simulink model "ctrl_student_HIL"  (R2015a)
settings: Solver=ode3  StartTime=0.0  StopTime=inf  FixedStep=0.01  RelTol=1e-3
undefined symbols (not defined in the file): DesiredPath, Elipscenter_radi, eta_dot_ini, K, K1, K2, l1, l2, l3, LAW, lim, lim_2, m, mu, pd, T_initialDP, U_ref
libraries: simulink x1
(part 3 of 4)

== system ctrl_student_HIL/tau to CSE mocell (only use for HIL testing) ==
  tau_d to model : Inport
  integrator reset : Inport  Port=2
  Constant : Constant  Value=eta_dot_ini(1)
  Constant1 : Constant  Value=eta_dot_ini(2)
  Constant2 : Constant  Value=eta_dot_ini(3)
  Demux : Demux  Outputs=3
  N_d : S-Function  Priority=2  FunctionName=NIVeriStandIO  Parameters=width dtype portnum stime stype btype  mask(NI VeriStand Outport){portnum=2, width=-1, stime=-1, dtype=auto, stype=auto, btype=0}
      mask prompts: portnum "Port number:"; width "Port dimensions (-1 for dynamically sized):"; stime "Sample time (-1 for inherited):"; dtype "Data type:"; stype "Signal type:"; btype "Block type:"
      mask help: Use this outport on any level of nested subsystems to allow NI VeriStand software to map signals to it.
      mask init:
      | NIVeriStandIO_init;
      settings: CopyFcn=NIVeriStand_MDL_functions('', 'IO_copy');  DeleteFcn=NIVeriStand_MDL_functions('', 'IO_delete');  MoveFcn=set_param(gcb, 'Mask', 'on');
      mask Callback portnum: NIVeriStand_MDL_functions('', 'IO_setportnum');
      mask TypeOptions dtype: auto | double | single | int8 | uint8 | int16 | uint16 | int32 | uint32 | boolean
      mask Callback dtype: NIVeriStand_MDL_functions('', 'IO_booleansignal');
      mask TypeOptions stype: auto | real | complex
      mask Display:
      | patch([-x x], [-y y], [.90980 .81960 .32156]);
      | plot([xrad -x x xrad], [yrad -y y yrad]);
      | fprintf('NI Out%d', portnum);
  X_d : S-Function  Priority=1  FunctionName=NIVeriStandIO  Parameters=width dtype portnum stime stype btype  mask(NI VeriStand Outport){portnum=1, width=-1, stime=-1, dtype=auto, stype=auto, btype=0}
      mask prompts: portnum "Port number:"; width "Port dimensions (-1 for dynamically sized):"; stime "Sample time (-1 for inherited):"; dtype "Data type:"; stype "Signal type:"; btype "Block type:"
      mask help: Use this outport on any level of nested subsystems to allow NI VeriStand software to map signals to it.
      mask init:
      | NIVeriStandIO_init;
      settings: CopyFcn=NIVeriStand_MDL_functions('', 'IO_copy');  DeleteFcn=NIVeriStand_MDL_functions('', 'IO_delete');  MoveFcn=set_param(gcb, 'Mask', 'on');
      mask Callback portnum: NIVeriStand_MDL_functions('', 'IO_setportnum');
      mask TypeOptions dtype: auto | double | single | int8 | uint8 | int16 | uint16 | int32 | uint32 | boolean
      mask Callback dtype: NIVeriStand_MDL_functions('', 'IO_booleansignal');
      mask TypeOptions stype: auto | real | complex
      mask Display:
      | patch([-x x], [-y y], [.90980 .81960 .32156]);
      | plot([xrad -x x xrad], [yrad -y y yrad]);
      | fprintf('NI Out%d', portnum);
  Y_d : S-Function  Priority=3  FunctionName=NIVeriStandIO  Parameters=width dtype portnum stime stype btype  mask(NI VeriStand Outport){portnum=3, width=-1, stime=-1, dtype=auto, stype=auto, btype=0}
      mask prompts: portnum "Port number:"; width "Port dimensions (-1 for dynamically sized):"; stime "Sample time (-1 for inherited):"; dtype "Data type:"; stype "Signal type:"; btype "Block type:"
      mask help: Use this outport on any level of nested subsystems to allow NI VeriStand software to map signals to it.
      mask init:
      | NIVeriStandIO_init;
      settings: CopyFcn=NIVeriStand_MDL_functions('', 'IO_copy');  DeleteFcn=NIVeriStand_MDL_functions('', 'IO_delete');  MoveFcn=set_param(gcb, 'Mask', 'on');
      mask Callback portnum: NIVeriStand_MDL_functions('', 'IO_setportnum');
      mask TypeOptions dtype: auto | double | single | int8 | uint8 | int16 | uint16 | int32 | uint32 | boolean
      mask Callback dtype: NIVeriStand_MDL_functions('', 'IO_booleansignal');
      mask TypeOptions stype: auto | real | complex
      mask Display:
      | patch([-x x], [-y y], [.90980 .81960 .32156]);
      | plot([xrad -x x xrad], [yrad -y y yrad]);
      | fprintf('NI Out%d', portnum);
  integrator reset model : S-Function  Priority=7  FunctionName=NIVeriStandIO  Parameters=width dtype portnum stime stype btype  mask(NI VeriStand Outport){portnum=7, width=-1, stime=-1, dtype=auto, stype=auto, btype=0}
      mask prompts: portnum "Port number:"; width "Port dimensions (-1 for dynamically sized):"; stime "Sample time (-1 for inherited):"; dtype "Data type:"; stype "Signal type:"; btype "Block type:"
      mask help: Use this outport on any level of nested subsystems to allow NI VeriStand software to map signals to it.
      mask init:
      | NIVeriStandIO_init;
      settings: CopyFcn=NIVeriStand_MDL_functions('', 'IO_copy');  DeleteFcn=NIVeriStand_MDL_functions('', 'IO_delete');  MoveFcn=set_param(gcb, 'Mask', 'on');
      mask Callback portnum: NIVeriStand_MDL_functions('', 'IO_setportnum');
      mask TypeOptions dtype: auto | double | single | int8 | uint8 | int16 | uint16 | int32 | uint32 | boolean
      mask Callback dtype: NIVeriStand_MDL_functions('', 'IO_booleansignal');
      mask TypeOptions stype: auto | real | complex
      mask Display:
      | patch([-x x], [-y y], [.90980 .81960 .32156]);
      | plot([xrad -x x xrad], [yrad -y y yrad]);
      | fprintf('NI Out%d', portnum);
  "psi_0 " : S-Function  Priority=4  FunctionName=NIVeriStandIO  Parameters=width dtype portnum stime stype btype  mask(NI VeriStand Outport){portnum=4, width=-1, stime=-1, dtype=auto, stype=auto, btype=0}
      mask prompts: portnum "Port number:"; width "Port dimensions (-1 for dynamically sized):"; stime "Sample time (-1 for inherited):"; dtype "Data type:"; stype "Signal type:"; btype "Block type:"
      mask help: Use this outport on any level of nested subsystems to allow NI VeriStand software to map signals to it.
      mask init:
      | NIVeriStandIO_init;
      settings: CopyFcn=NIVeriStand_MDL_functions('', 'IO_copy');  DeleteFcn=NIVeriStand_MDL_functions('', 'IO_delete');  MoveFcn=set_param(gcb, 'Mask', 'on');
      mask Callback portnum: NIVeriStand_MDL_functions('', 'IO_setportnum');
      mask TypeOptions dtype: auto | double | single | int8 | uint8 | int16 | uint16 | int32 | uint32 | boolean
      mask Callback dtype: NIVeriStand_MDL_functions('', 'IO_booleansignal');
      mask TypeOptions stype: auto | real | complex
      mask Display:
      | patch([-x x], [-y y], [.90980 .81960 .32156]);
      | plot([xrad -x x xrad], [yrad -y y yrad]);
      | fprintf('NI Out%d', portnum);
  x_0 : S-Function  Priority=5  FunctionName=NIVeriStandIO  Parameters=width dtype portnum stime stype btype  mask(NI VeriStand Outport){portnum=5, width=-1, stime=-1, dtype=auto, stype=auto, btype=0}
      mask prompts: portnum "Port number:"; width "Port dimensions (-1 for dynamically sized):"; stime "Sample time (-1 for inherited):"; dtype "Data type:"; stype "Signal type:"; btype "Block type:"
      mask help: Use this outport on any level of nested subsystems to allow NI VeriStand software to map signals to it.
      mask init:
      | NIVeriStandIO_init;
      settings: CopyFcn=NIVeriStand_MDL_functions('', 'IO_copy');  DeleteFcn=NIVeriStand_MDL_functions('', 'IO_delete');  MoveFcn=set_param(gcb, 'Mask', 'on');
      mask Callback portnum: NIVeriStand_MDL_functions('', 'IO_setportnum');
      mask TypeOptions dtype: auto | double | single | int8 | uint8 | int16 | uint16 | int32 | uint32 | boolean
      mask Callback dtype: NIVeriStand_MDL_functions('', 'IO_booleansignal');
      mask TypeOptions stype: auto | real | complex
      mask Display:
      | patch([-x x], [-y y], [.90980 .81960 .32156]);
      | plot([xrad -x x xrad], [yrad -y y yrad]);
      | fprintf('NI Out%d', portnum);
  y_0 : S-Function  Priority=6  FunctionName=NIVeriStandIO  Parameters=width dtype portnum stime stype btype  mask(NI VeriStand Outport){portnum=6, width=-1, stime=-1, dtype=auto, stype=auto, btype=0}
      mask prompts: portnum "Port number:"; width "Port dimensions (-1 for dynamically sized):"; stime "Sample time (-1 for inherited):"; dtype "Data type:"; stype "Signal type:"; btype "Block type:"
      mask help: Use this outport on any level of nested subsystems to allow NI VeriStand software to map signals to it.
      mask init:
      | NIVeriStandIO_init;
      settings: CopyFcn=NIVeriStand_MDL_functions('', 'IO_copy');  DeleteFcn=NIVeriStand_MDL_functions('', 'IO_delete');  MoveFcn=set_param(gcb, 'Mask', 'on');
      mask Callback portnum: NIVeriStand_MDL_functions('', 'IO_setportnum');
      mask TypeOptions dtype: auto | double | single | int8 | uint8 | int16 | uint16 | int32 | uint32 | boolean
      mask Callback dtype: NIVeriStand_MDL_functions('', 'IO_booleansignal');
      mask TypeOptions stype: auto | real | complex
      mask Display:
      | patch([-x x], [-y y], [.90980 .81960 .32156]);
      | plot([xrad -x x xrad], [yrad -y y yrad]);
      | fprintf('NI Out%d', portnum);
  wires:
  tau_d to model/1 -> Demux/1
  Demux/1 -> X_d/1
  Demux/2 -> Y_d/1
  Demux/3 -> N_d/1
  Constant2/1 -> "psi_0 "/1
  Constant1/1 -> y_0/1
  Constant/1 -> x_0/1
  integrator reset/1 -> integrator reset model/1

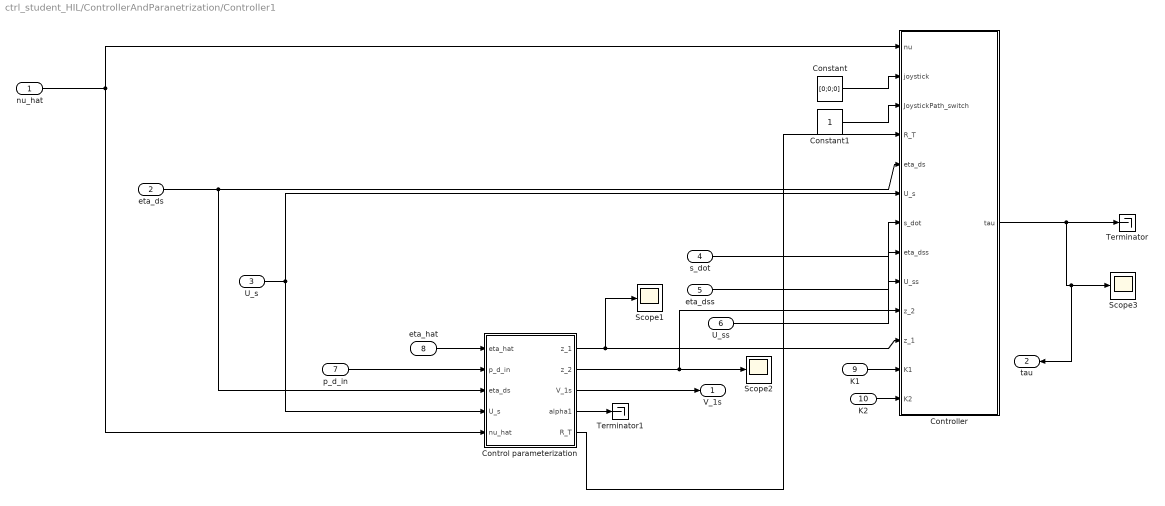
== system ctrl_student_HIL/ControllerAndParanetrization/Controller1 ==
  nu_hat : Inport
  "eta_ds " : Inport  Port=2
  U_s : Inport  Port=3
  s_dot : Inport  Port=4
  eta_dss : Inport  Port=5
  U_ss : Inport  Port=6
  p_d_in : Inport  Port=7
  eta_hat : Inport  Port=8
  K1 : Inport  Port=9
  K2 : Inport  Port=10
  Constant : Constant  Value=[0;0;0]
  Constant1 : Constant
  Control parameterization : Subsystem
  Controller : Subsystem
  Scope1 : Scope
      settings: YMin=-6.76763  YMax=7.09799  SaveName=ScopeData8
  Scope2 : Scope
  Scope3 : Scope
      settings: YMin=-11.79233  YMax=2.58486  SaveName=ScopeData3
  Terminator : Terminator
  Terminator1 : Terminator
  "V_1s " : Outport
  tau : Outport  Port=2
  wires:
  Control parameterization/1(z_1) -> Scope1/1, Controller/11(z_1)
  Control parameterization/2(z_2) -> Scope2/1, Controller/10(z_2)
  nu_hat/1 -> Controller/1(" nu"), Control parameterization/5(nu_hat)
  Control parameterization/5("R_T ") -> Controller/4(R_T)
  Constant/1 -> Controller/2(joystick)
  Constant1/1 -> Controller/3(JoystickPath_switch)
  Controller/1(tau) -> tau/1, Scope3/1, Terminator/1
  Control parameterization/4(alpha1) -> Terminator1/1
  U_ss/1 -> Controller/9(U_ss)
  s_dot/1 -> Controller/7(s_dot)
  eta_dss/1 -> Controller/8(eta_dss)
  Control parameterization/3("V_1s ") -> "V_1s "/1
  U_s/1 -> Controller/6(U_s), Control parameterization/4(U_s)
  "eta_ds "/1 -> Control parameterization/3("eta_ds "), Controller/5(eta_ds)
  p_d_in/1 -> Control parameterization/2("p_d_in ")
  eta_hat/1 -> Control parameterization/1(eta_hat)
  K1/1 -> Controller/12(K1)
  K2/1 -> Controller/13(K2)

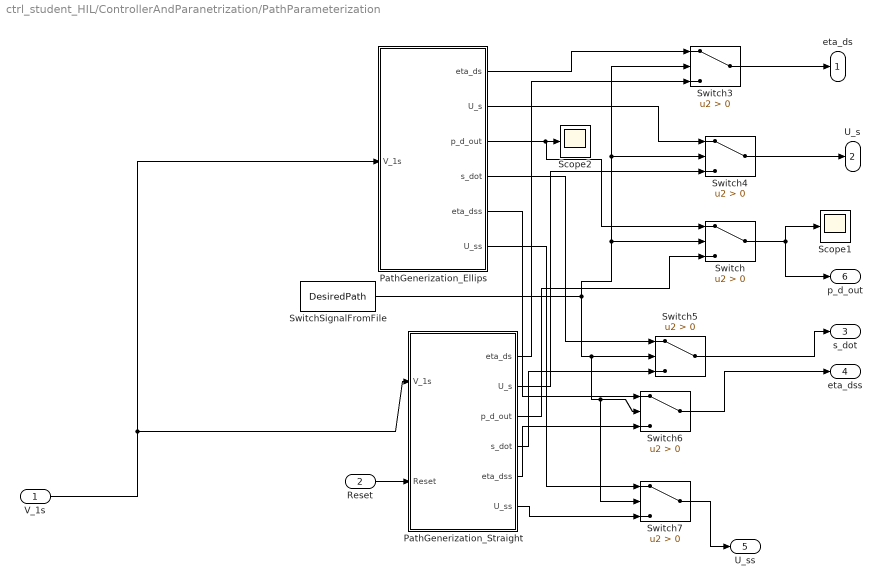
== system ctrl_student_HIL/ControllerAndParanetrization/PathParameterization ==
  V_1s : Inport
  "Reset " : Inport  Port=2
  PathGenerization_Ellips : Subsystem
  PathGenerization_Straight : Subsystem
  Scope1 : Scope
      settings: YMin=-1.25  YMax=11.25  SaveName=ScopeData2
  Scope2 : Scope
      settings: YMin=-4.75  YMax=12.75  SaveName=ScopeData12
  Switch{,3..7} (6 alike) : Switch  Criteria=u2 > Threshold
  SwitchSignalFromFile : Constant  Value=DesiredPath
  eta_ds : Outport
  U_s : Outport  Port=2
  s_dot : Outport  Port=3
  eta_dss : Outport  Port=4
  U_ss : Outport  Port=5
  p_d_out : Outport  Port=6
  wires:
  PathGenerization_Ellips/4(s_dot) -> Switch5/1
  PathGenerization_Straight/4(s_dot) -> Switch5/3
  PathGenerization_Ellips/6(U_ss) -> Switch7/1
  PathGenerization_Straight/6(U_ss) -> Switch7/3
  PathGenerization_Straight/5("eta_dss ") -> Switch6/3
  PathGenerization_Straight/1(eta_ds) -> Switch3/3
  PathGenerization_Ellips/1(eta_ds) -> Switch3/1
  PathGenerization_Straight/2(U_s) -> Switch4/3
  PathGenerization_Straight/3(p_d_out) -> Switch/3
  PathGenerization_Ellips/2(U_s) -> Switch4/1
  PathGenerization_Ellips/3(p_d_out) -> Switch/1, Scope2/1
  SwitchSignalFromFile/1 -> Switch4/2, Switch3/2, Switch/2, Switch7/2, Switch6/2, Switch5/2
  Switch3/1 -> eta_ds/1
  Switch4/1 -> U_s/1
  Switch5/1 -> s_dot/1
  Switch6/1 -> eta_dss/1
  Switch7/1 -> U_ss/1
  V_1s/1 -> PathGenerization_Ellips/1(V_1s), PathGenerization_Straight/1(V_1s)
  Switch/1 -> p_d_out/1, Scope1/1
  PathGenerization_Ellips/5("eta_dss ") -> Switch6/1
  "Reset "/1 -> PathGenerization_Straight/2("Reset ")

== system ctrl_student_HIL/DPObserver1/Bias ==
  eta : Inport
  etaHat : Inport  Port=2
  L3 : Inport  Port=3
  biasOffset : Inport  Port=4  PortDimensions=1
  Constant : Constant  Value=[1;1;1]
  IC1 : InitialCondition  Value=[0;0;0]
  Product : Product
  Reshape1 : Reshape  OutputDimensionality=Customize  OutputDimensions=[3,1]
  Sum : Sum  Inputs=|++
  bHat : Integrator
  bHatDot : MATLAB Function  TreatAsAtomicUnit=on
  bias : Outport
  wires:
  bHatDot/1(bHatDot) -> bHat/1
  eta/1 -> bHatDot/2(eta)
  etaHat/1 -> bHatDot/3(etaHat)
  L3/1 -> bHatDot/1(L3)
  IC1/1 -> bias/1
  Sum/1 -> IC1/1
  biasOffset/1 -> Product/1
  Product/1 -> Reshape1/1
  Constant/1 -> Product/2
  bHat/1 -> Sum/1
  Reshape1/1 -> Sum/2

== system ctrl_student_HIL/DPObserver1/Subsystem ==
  bHat : Inport
  D : Inport  Port=2
  tau : Inport  Port=3
  eta : Inport  Port=4
  etaHat : Inport  Port=5
  R : Inport  Port=6
  L2 : Inport  Port=7
  IC : InitialCondition  Value=[0;0;0]
  M : MATLAB Function  TreatAsAtomicUnit=on
  nuHat : Integrator  InitialCondition=[0;0;0]
  nuHatDot : MATLAB Function  TreatAsAtomicUnit=on
  nu : Outport
  wires:
  tau/1 -> nuHatDot/6(tau)
  bHat/1 -> nuHatDot/2(bHat)
  M/1(M) -> nuHatDot/4(M)
  nuHat/1 -> nuHatDot/1(nuHat), nu/1
  etaHat/1 -> nuHatDot/9(etaHat)
  R/1 -> nuHatDot/8(R)
  eta/1 -> nuHatDot/7(eta)
  nuHatDot/1(nuHatDot) -> IC/1
  D/1 -> nuHatDot/3(D)
  L2/1 -> nuHatDot/5(L2)
  IC/1 -> nuHat/1

== system ctrl_student_HIL/DPObserver1/etaHat ==
  nuHat : Inport
  etaHatInn : Inport  Port=2
  etaInn : Inport  Port=3
  R : Inport  Port=4
  L1 : Inport  Port=5
  PosReset : Inport  Port=6
  Reshape1 : Reshape  OutputDimensionality=Customize  OutputDimensions=[3,3]
  Reshape3 : Reshape  OutputDimensionality=Customize  OutputDimensions=[3,1]
  etaHat : Integrator  ExternalReset=rising  InitialCondition=[0;0;0]
  etaHatDot : MATLAB Function  TreatAsAtomicUnit=on
  etaHatDotOut : Outport
  etaHatOut : Outport  Port=2
  wires:
  etaHat/1 -> etaHatOut/1
  etaHatDot/1(etaHatDot) -> etaHat/1, etaHatDotOut/1
  L1/1 -> etaHatDot/3(L1)
  R/1 -> Reshape1/1
  nuHat/1 -> Reshape3/1
  etaInn/1 -> etaHatDot/4(eta)
  etaHatInn/1 -> etaHatDot/1(etaHat)
  Reshape3/1 -> etaHatDot/2(nuHat)
  Reshape1/1 -> etaHatDot/5(R)
  PosReset/1 -> etaHat/2

== system ctrl_student_HIL/Noise generator/Downsample	signal ==
  sampling frequency : Inport
  step size : Inport  Port=2
  MATLAB Function : MATLAB Function  TreatAsAtomicUnit=on
  counter : Memory
  trigger : Outport
  wires:
  sampling frequency/1 -> MATLAB Function/1(f)
  step size/1 -> MATLAB Function/2(h)
  counter/1 -> MATLAB Function/3(i)
  MATLAB Function/1(count) -> counter/1, trigger/1

== system ctrl_student_HIL/Noise generator/Sample & hold ==
  trigger : Inport
  input : Inport  Port=2
  Hold : Memory
  MATLAB Function1 : MATLAB Function  TreatAsAtomicUnit=on
  output : Outport
  wires:
  MATLAB Function1/1(output) -> output/1, Hold/1
  trigger/1 -> MATLAB Function1/1(counter)
  input/1 -> MATLAB Function1/2(input)
  Hold/1 -> MATLAB Function1/3(hold)

== system ctrl_student_HIL/Noise generator/noise generator ==
  step size : Inport
  noise power position : Inport  Port=2
  noise power heading : Inport  Port=3
  Band-limited white noise psi : Subsystem
  Band-limited white noise x : Subsystem
  Band-limited white noise y : Subsystem
  Mux1 : Mux  Inputs=3
  Out1 : Outport
  wires:
  Mux1/1 -> Out1/1
  step size/1 -> Band-limited white noise x/1(step size), Band-limited white noise psi/1(step size), Band-limited white noise y/1(step size)
  noise power position/1 -> Band-limited white noise y/2(power), Band-limited white noise x/2(power)
  Band-limited white noise x/1(noise) -> Mux1/1
  Band-limited white noise y/1(noise) -> Mux1/2
  Band-limited white noise psi/1(noise) -> Mux1/3
  noise power heading/1 -> Band-limited white noise psi/2(power)

== system ctrl_student_HIL/ControllerAndParanetrization/Controller1/Control parameterization ==
  eta_hat : Inport
  "p_d_in " : Inport  Port=2
  "eta_ds " : Inport  Port=3
  U_s : Inport  Port=4
  nu_hat : Inport  Port=5
  "BacksteppingParameterization " : Subsystem
  z_1 : Outport
  z_2 : Outport  Port=2
  "V_1s " : Outport  Port=3
  alpha1 : Outport  Port=4
  "R_T " : Outport  Port=5
  wires:
  "eta_ds "/1 -> "BacksteppingParameterization "/3(eta_ds)
  eta_hat/1 -> "BacksteppingParameterization "/1(eta_hat)
  "p_d_in "/1 -> "BacksteppingParameterization "/2("p_d_in ")
  "BacksteppingParameterization "/1(V_1s_out) -> "V_1s "/1
  U_s/1 -> "BacksteppingParameterization "/4(U_s)
  "BacksteppingParameterization "/3(z_2) -> z_2/1
  nu_hat/1 -> "BacksteppingParameterization "/5(nu_hat)
  "BacksteppingParameterization "/2(z_1) -> z_1/1
  "BacksteppingParameterization "/4("alpha1 ") -> alpha1/1
  "BacksteppingParameterization "/5(R_T) -> "R_T "/1

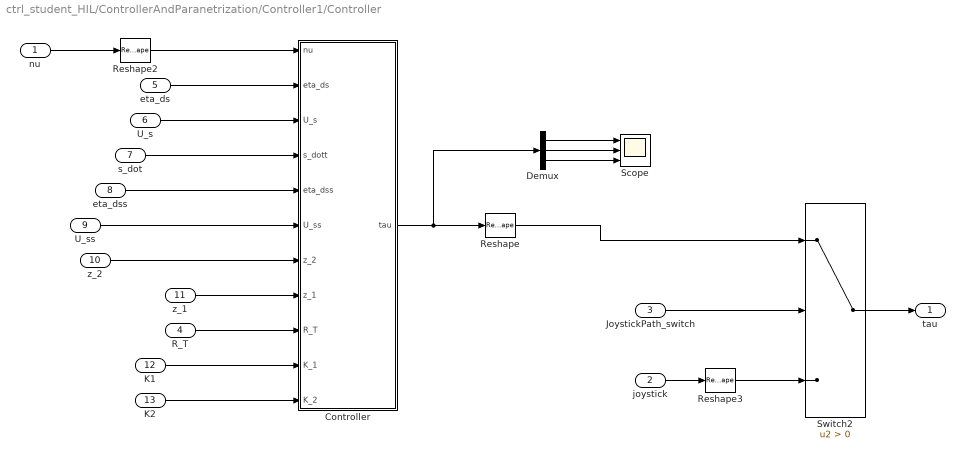
== system ctrl_student_HIL/ControllerAndParanetrization/Controller1/Controller ==
  " nu" : Inport
  joystick : Inport  Port=2
  JoystickPath_switch : Inport  Port=3
  R_T : Inport  Port=4
  eta_ds : Inport  Port=5
  U_s : Inport  Port=6
  s_dot : Inport  Port=7
  eta_dss : Inport  Port=8
  U_ss : Inport  Port=9
  z_2 : Inport  Port=10
  z_1 : Inport  Port=11
  K1 : Inport  Port=12
  K2 : Inport  Port=13
  Controller : Subsystem
  Demux : Demux  Outputs=3
  Reshape : Reshape  OutputDimensionality=Customize  OutputDimensions=[3,1]
  Reshape2 : Reshape  OutputDimensionality=Customize  OutputDimensions=[3,1]
  Reshape3 : Reshape  OutputDimensionality=Customize  OutputDimensions=[3,1]
  Scope : Scope  NumInputPorts=3
      settings: YMin=-1.81121~-0.05182~-0.00671  YMax=5.53458~0.46636~0.06037  SaveName=ScopeData6
  Switch2 : Switch  Criteria=u2 > Threshold
  tau : Outport
  wires:
  " nu"/1 -> Reshape2/1
  Switch2/1 -> tau/1
  joystick/1 -> Reshape3/1
  JoystickPath_switch/1 -> Switch2/2
  eta_ds/1 -> Controller/2(eta_ds)
  U_s/1 -> Controller/3(U_s)
  s_dot/1 -> Controller/4(s_dott)
  eta_dss/1 -> Controller/5(eta_dss)
  U_ss/1 -> Controller/6(U_ss)
  Controller/1(tau) -> Demux/1, Reshape/1
  R_T/1 -> Controller/9(R_T)
  K1/1 -> Controller/10(K_1)
  K2/1 -> Controller/11(K_2)
  Reshape/1 -> Switch2/1
  z_2/1 -> Controller/7(z_2)
  Reshape2/1 -> Controller/1(nu)
  Reshape3/1 -> Switch2/3
  z_1/1 -> Controller/8(z_1)
  Demux/1 -> Scope/1
  Demux/2 -> Scope/2
  Demux/3 -> Scope/3

== system ctrl_student_HIL/ControllerAndParanetrization/PathParameterization/PathGenerization_Ellips ==
  V_1s : Inport
  Check_s : Subsystem
  IC : InitialCondition  Value=0
  Memory : Memory
  "Path parametization " : Subsystem
  Scope3 : Scope  NumInputPorts=2
      settings: YMin=-0.125  YMax=1.12502  SaveName=ScopeData13
  Scope4 : Scope
  parameter generator : Subsystem
  eta_ds : Outport
  U_s : Outport  Port=2
  p_d_out : Outport  Port=3
  s_dot : Outport  Port=4
  "eta_dss " : Outport  Port=5
  U_ss : Outport  Port=6
  wires:
  "Path parametization "/1("p_d_out ") -> p_d_out/1
  parameter generator/1(s) -> Scope3/1, Check_s/1(s_inn)
  "Path parametization "/4(p_d_sdott) -> parameter generator/2(p_d_sdott)
  parameter generator/2(U_s) -> U_s/1
  "Path parametization "/2("eta_ds ") -> parameter generator/3(eta_ds), eta_ds/1
  V_1s/1 -> parameter generator/1(V_1s)
  Check_s/1(s_out) -> Scope4/1, Scope3/2, "Path parametization "/1(s)
  Check_s/2(U_ref) -> IC/1
  IC/1 -> "Path parametization "/2(U_ref), parameter generator/4(U_ref)
  Memory/1 -> parameter generator/5(SwitchSignal)
  Check_s/3(SwitchSignal) -> Memory/1
  parameter generator/3("s_dot ") -> s_dot/1
  "Path parametization "/3(eta_dss) -> "eta_dss "/1
  "Path parametization "/5(U_ss) -> U_ss/1

== system ctrl_student_HIL/ControllerAndParanetrization/PathParameterization/PathGenerization_Straight ==
  V_1s : Inport
  "Reset " : Inport  Port=2
  IC : InitialCondition  Value=0
  Memory : Memory
  "Path parametization " : Subsystem
  Scope1 : Scope
  Scope3 : Scope
  parameter generator : Subsystem
  eta_ds : Outport
  U_s : Outport  Port=2
  p_d_out : Outport  Port=3
  s_dot : Outport  Port=4
  "eta_dss " : Outport  Port=5
  U_ss : Outport  Port=6
  wires:
  "Path parametization "/1("p_d_out ") -> p_d_out/1
  "Path parametization "/3(p_d_sdott) -> parameter generator/2(p_d_sdott)
  "Path parametization "/2("eta_ds ") -> parameter generator/3(eta_ds), eta_ds/1
  V_1s/1 -> parameter generator/1(V_1s)
  parameter generator/1(s) -> Scope3/1, "Path parametization "/1(s)
  IC/1 -> parameter generator/4(U_ref)
  Memory/1 -> parameter generator/5(SwitchSignal)
  "Path parametization "/4(SwitchSignal) -> Memory/1
  parameter generator/3("s_dot ") -> s_dot/1
  "Path parametization "/5(eta_dss) -> "eta_dss "/1
  "Path parametization "/6(U_ss) -> U_ss/1
  parameter generator/2(U_s) -> Scope1/1, U_s/1
  "Path parametization "/7(U) -> IC/1
  "Reset "/1 -> "Path parametization "/2("Reset ")

== system ctrl_student_HIL/Noise generator/noise generator/Band-limited white noise psi ==
  step size : Inport
  power : Inport  Port=2
  Divide : Product  Inputs=*/
  Product : Product
  Sqrt : Sqrt  SaturateOnIntegerOverflow=on
  White Noise : RandomNumber  DisableCoverage=on  Seed=9025
  noise : Outport
  wires:
  White Noise/1 -> Product/2
  Product/1 -> noise/1
  step size/1 -> Divide/2
  Divide/1 -> Sqrt/1
  Sqrt/1 -> Product/1
  power/1 -> Divide/1

== system ctrl_student_HIL/Noise generator/noise generator/Band-limited white noise x ==
  step size : Inport
  power : Inport  Port=2
  Divide : Product  Inputs=*/
  Product : Product
  Sqrt : Sqrt  SaturateOnIntegerOverflow=on
  White Noise : RandomNumber  DisableCoverage=on  Seed=9024
  noise : Outport
  wires:
  White Noise/1 -> Product/2
  Product/1 -> noise/1
  step size/1 -> Divide/2
  Divide/1 -> Sqrt/1
  Sqrt/1 -> Product/1
  power/1 -> Divide/1

== system ctrl_student_HIL/Noise generator/noise generator/Band-limited white noise y ==
  step size : Inport
  power : Inport  Port=2
  Divide : Product  Inputs=*/
  Product : Product
  Sqrt : Sqrt  SaturateOnIntegerOverflow=on
  White Noise : RandomNumber  DisableCoverage=on  Seed=123
  noise : Outport
  wires:
  White Noise/1 -> Product/2
  Product/1 -> noise/1
  step size/1 -> Divide/2
  Divide/1 -> Sqrt/1
  Sqrt/1 -> Product/1
  power/1 -> Divide/1

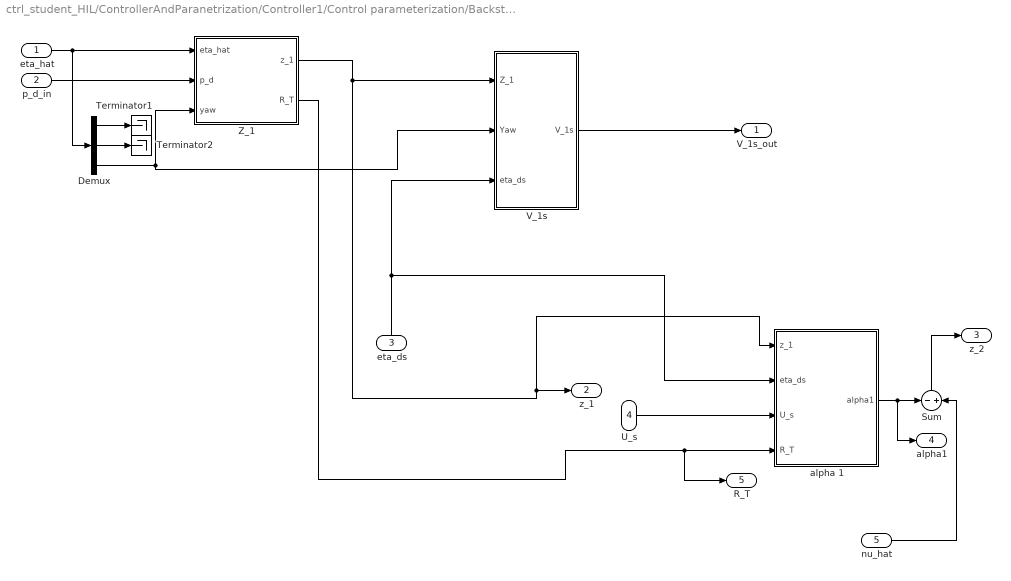
== system ctrl_student_HIL/ControllerAndParanetrization/Controller1/Control parameterization/BacksteppingParameterization  ==
  eta_hat : Inport
  "p_d_in " : Inport  Port=2
  eta_ds : Inport  Port=3
  U_s : Inport  Port=4
  nu_hat : Inport  Port=5
  Demux : Demux  Outputs=3
  Sum : Sum  Inputs=-|+
  Terminator1 : Terminator
  Terminator2 : Terminator
  V_1s : Subsystem
  Z_1 : Subsystem
  alpha 1 : Subsystem
  V_1s_out : Outport
  z_1 : Outport  Port=2
  z_2 : Outport  Port=3
  "alpha1 " : Outport  Port=4
  R_T : Outport  Port=5
  wires:
  eta_ds/1 -> alpha 1/2(eta_ds), V_1s/3(eta_ds)
  eta_hat/1 -> Demux/1, Z_1/1(eta_hat)
  "p_d_in "/1 -> Z_1/2(p_d)
  Demux/3 -> V_1s/2(Yaw), Z_1/3("yaw ")
  V_1s/1(V_1s) -> V_1s_out/1
  alpha 1/1(alpha1) -> "alpha1 "/1, Sum/1
  U_s/1 -> alpha 1/3(U_s)
  Z_1/1(z_1) -> alpha 1/1(z_1), z_1/1, V_1s/1(Z_1)
  Z_1/2(R_T) -> R_T/1, alpha 1/4(R_T)
  nu_hat/1 -> Sum/2
  Sum/1 -> z_2/1
  Demux/1 -> Terminator1/1
  Demux/2 -> Terminator2/1

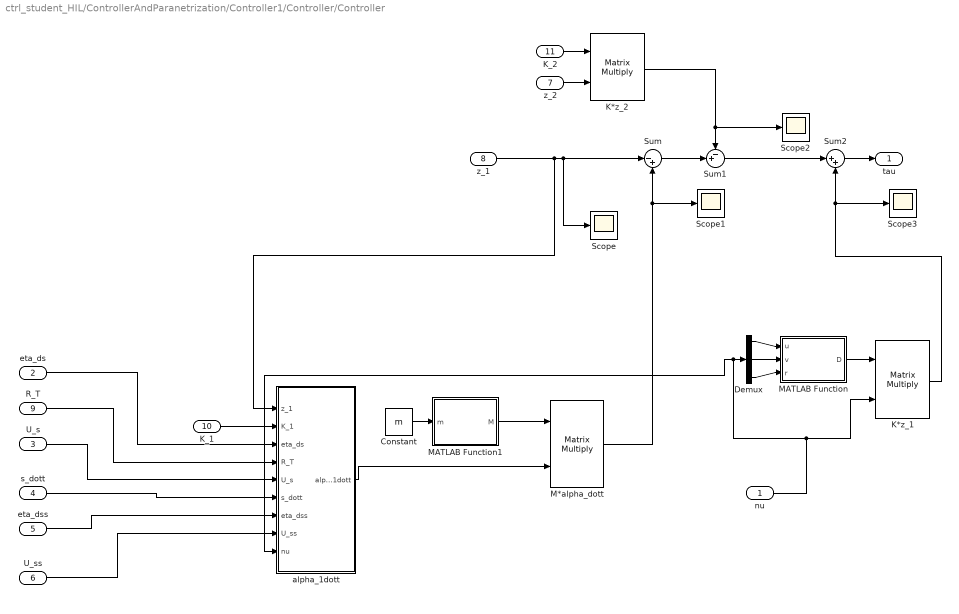
== system ctrl_student_HIL/ControllerAndParanetrization/Controller1/Controller/Controller ==
  nu : Inport
  eta_ds : Inport  Port=2
  U_s : Inport  Port=3
  s_dott : Inport  Port=4
  eta_dss : Inport  Port=5
  U_ss : Inport  Port=6
  z_2 : Inport  Port=7
  z_1 : Inport  Port=8
  R_T : Inport  Port=9
  K_1 : Inport  Port=10
  K_2 : Inport  Port=11
  Constant : Constant  Value=m
  Demux : Demux  Outputs=3
  K*z_1 : Product  Multiplication=Matrix(*)
  K*z_2 : Product  Multiplication=Matrix(*)
  M*alpha_dott : Product  Multiplication=Matrix(*)
  MATLAB Function : MATLAB Function  TreatAsAtomicUnit=on
  MATLAB Function1 : MATLAB Function  TreatAsAtomicUnit=on
  Scope{,1..3} (4 alike) : Scope
      Scope settings: YMin=-1.86769  YMax=9.78914
      Scope1 settings: YMin=-0.31241  YMax=0.96684  SaveName=ScopeData2
      Scope2 settings: YMin=-1.22848  YMax=2.91428  SaveName=ScopeData3
      Scope3 settings: YMin=-1.62155  YMax=0.35636  SaveName=ScopeData4
  Sum : Sum  Inputs=|-+
  Sum1 : Sum  Inputs=-+|
  Sum2 : Sum  Inputs=|++
  alpha_1dott : Subsystem
  tau : Outport
  wires:
  alpha_1dott/1(alpha_1dott) -> M*alpha_dott/2
  MATLAB Function1/1(M) -> M*alpha_dott/1
  z_1/1 -> alpha_1dott/1(z_1), Scope/1, Sum/1
  Sum/1 -> Sum1/2
  Sum1/1 -> Sum2/1
  Sum2/1 -> tau/1
  z_2/1 -> K*z_2/2
  K*z_1/1 -> Sum2/2, Scope3/1
  nu/1 -> alpha_1dott/9(nu), Demux/1, K*z_1/2
  eta_ds/1 -> alpha_1dott/3(eta_ds)
  R_T/1 -> alpha_1dott/4(R_T)
  U_s/1 -> alpha_1dott/5(U_s)
  s_dott/1 -> alpha_1dott/6(s_dott)
  eta_dss/1 -> alpha_1dott/7(eta_dss)
  U_ss/1 -> alpha_1dott/8(U_ss)
  K_1/1 -> alpha_1dott/2(K_1)
  K_2/1 -> K*z_2/1
  Demux/1 -> MATLAB Function/1(u)
  Demux/2 -> MATLAB Function/2(v)
  Demux/3 -> MATLAB Function/3(r)
  MATLAB Function/1(D) -> K*z_1/1
  Constant/1 -> MATLAB Function1/1(m)
  K*z_2/1 -> Scope2/1, Sum1/1
  M*alpha_dott/1 -> Scope1/1, Sum/2

== system ctrl_student_HIL/ControllerAndParanetrization/PathParameterization/PathGenerization_Ellips/Check_s ==
  s_inn : Inport
  CheckS&getU : MATLAB Function  TreatAsAtomicUnit=on
  Constant : Constant  Value=U_ref
  s_out : Outport
  U_ref : Outport  Port=2
  SwitchSignal : Outport  Port=3
  wires:
  CheckS&getU/1(s_out) -> s_out/1
  s_inn/1 -> CheckS&getU/1(s_inn)
  CheckS&getU/2(U) -> U_ref/1
  Constant/1 -> CheckS&getU/2(U_ref)
  CheckS&getU/3(Switch) -> SwitchSignal/1

== system ctrl_student_HIL/ControllerAndParanetrization/PathParameterization/PathGenerization_Ellips/Path parametization  ==
  s : Inport
  U_ref : Inport  Port=2
  Elipscenter_radi : Constant  Value=Elipscenter_radi  VectorParams1D=off
  Subsystem : Subsystem
  "p_d_out " : Outport
  "eta_ds " : Outport  Port=2
  eta_dss : Outport  Port=3
  p_d_sdott : Outport  Port=4
  U_ss : Outport  Port=5
  wires:
  Elipscenter_radi/1 -> Subsystem/1(Elipscenter_radi)
  s/1 -> Subsystem/2(s)
  Subsystem/1(P_d) -> "p_d_out "/1
  Subsystem/2(Pd_s) -> p_d_sdott/1
  Subsystem/3(eta_ds) -> "eta_ds "/1
  Subsystem/4(eta_dss) -> eta_dss/1
  U_ref/1 -> Subsystem/3(U_ref)
  Subsystem/5(U_ss) -> U_ss/1

== system ctrl_student_HIL/ControllerAndParanetrization/PathParameterization/PathGenerization_Ellips/parameter generator ==
  V_1s : Inport
  p_d_sdott : Inport  Port=2
  eta_ds : Inport  Port=3
  U_ref : Inport  Port=4
  SwitchSignal : Inport  Port=5
  Integrator : Integrator  ExternalReset=rising
  MATLAB Function1 : MATLAB Function  TreatAsAtomicUnit=on
  TASK : Constant  Value=LAW
  UpdateLaw : MATLAB Function  TreatAsAtomicUnit=on
  "mu " : Constant  Value=mu
  s : Outport
  U_s : Outport  Port=2
  "s_dot " : Outport  Port=3
  wires:
  Integrator/1 -> s/1
  p_d_sdott/1 -> UpdateLaw/1(p_d_sdot)
  UpdateLaw/1(s_dot) -> "s_dot "/1, Integrator/1
  UpdateLaw/2(U_s) -> U_s/1
  U_ref/1 -> UpdateLaw/2(U_ref)
  V_1s/1 -> UpdateLaw/3(V_1s)
  "mu "/1 -> UpdateLaw/4(mu)
  eta_ds/1 -> UpdateLaw/5(eta_ds)
  MATLAB Function1/1(SwitchSignal_Out) -> Integrator/2
  TASK/1 -> UpdateLaw/6(LAW)
  SwitchSignal/1 -> MATLAB Function1/1(SwitchSignal_In)

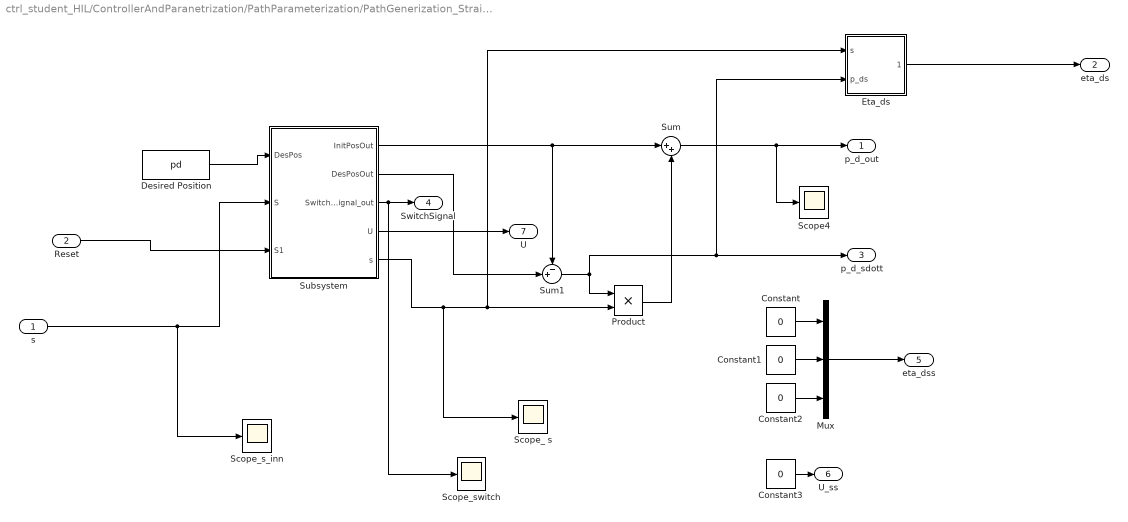
== system ctrl_student_HIL/ControllerAndParanetrization/PathParameterization/PathGenerization_Straight/Path parametization  ==
  s : Inport
  "Reset " : Inport  Port=2
  Constant{,1..3} (4 alike) : Constant  Value=0
  Desired Position : Constant  Value=pd  VectorParams1D=off
  Eta_ds : Subsystem
  Mux : Mux  Inputs=3
  Product : Product
  Scope4 : Scope
      settings: YMin=0  YMax=12
  Scope_ s : Scope
      settings: YMin=0  YMax=1
  Scope_s_inn : Scope
      settings: TimeRange=1000  YMin=0  YMax=1.4
  Scope_switch : Scope
      settings: YMin=-0  YMax=2
  Subsystem : Subsystem
  Sum : Sum  Inputs=|++
  Sum1 : Sum  Inputs=-+|
  "p_d_out " : Outport
  "eta_ds " : Outport  Port=2
  p_d_sdott : Outport  Port=3
  SwitchSignal : Outport  Port=4
  eta_dss : Outport  Port=5
  U_ss : Outport  Port=6
  U : Outport  Port=7
  wires:
  Product/1 -> Sum/2
  Desired Position/1 -> Subsystem/1(DesPos)
  s/1 -> Scope_s_inn/1, Subsystem/2(S)
  Sum1/1 -> Product/1, Eta_ds/2(p_ds), p_d_sdott/1
  Eta_ds/1(eta_ds) -> "eta_ds "/1
  Subsystem/1(InitPosOut) -> Sum1/1, Sum/1
  Subsystem/3(SwitchSignal_out) -> Scope_switch/1, SwitchSignal/1
  Subsystem/2(DesPosOut) -> Sum1/2
  Sum/1 -> Scope4/1, "p_d_out "/1
  Mux/1 -> eta_dss/1
  Constant/1 -> Mux/1
  Constant1/1 -> Mux/2
  Constant2/1 -> Mux/3
  Constant3/1 -> U_ss/1
  Subsystem/4(U) -> U/1
  Subsystem/5(s) -> Scope_ s/1, Eta_ds/1(s), Product/2
  "Reset "/1 -> Subsystem/3(S1)

== system ctrl_student_HIL/ControllerAndParanetrization/PathParameterization/PathGenerization_Straight/parameter generator ==
  V_1s : Inport
  p_d_sdott : Inport  Port=2
  eta_ds : Inport  Port=3
  U_ref : Inport  Port=4
  SwitchSignal : Inport  Port=5
  Integrator : Integrator  ExternalReset=rising
  MATLAB Function1 : MATLAB Function  TreatAsAtomicUnit=on
  TASK : Constant  Value=LAW
  UpdateLaw : MATLAB Function  TreatAsAtomicUnit=on
  "mu " : Constant  Value=mu
  s : Outport
  U_s : Outport  Port=2
  "s_dot " : Outport  Port=3
  wires:
  Integrator/1 -> s/1
  p_d_sdott/1 -> UpdateLaw/1(p_d_sdot)
  UpdateLaw/1(s_dot) -> "s_dot "/1, Integrator/1
  UpdateLaw/2(U_s) -> U_s/1
  U_ref/1 -> UpdateLaw/2(U_ref)
  V_1s/1 -> UpdateLaw/3(V_1s)
  "mu "/1 -> UpdateLaw/4(mu)
  eta_ds/1 -> UpdateLaw/5(eta_ds)
  MATLAB Function1/1(SwitchSignal_Out) -> Integrator/2
  TASK/1 -> UpdateLaw/6(LAW)
  SwitchSignal/1 -> MATLAB Function1/1(SwitchSignal_In)

== system ctrl_student_HIL/ControllerAndParanetrization/Controller1/Control parameterization/BacksteppingParameterization /V_1s ==
  Z_1 : Inport
  Yaw : Inport  Port=2
  eta_ds : Inport  Port=3
  Gain : Gain  Gain=-1
  MATLAB Function : MATLAB Function  TreatAsAtomicUnit=on
  MATLAB Function1 : MATLAB Function  TreatAsAtomicUnit=on
  Product : Product  Multiplication=Matrix(*)
  Product1 : Product  Multiplication=Matrix(*)
  Rotation Matrix : MATLAB Function  TreatAsAtomicUnit=on
  V_1s : Outport
  wires:
  Z_1/1 -> MATLAB Function/1(z_1)
  Rotation Matrix/1(R) -> MATLAB Function1/1(R)
  MATLAB Function1/1(R_T) -> Product/2
  Yaw/1 -> Rotation Matrix/1(yaw)
  MATLAB Function/1(z_1T) -> Product/1
  Product/1 -> Product1/1
  Product1/1 -> Gain/1
  eta_ds/1 -> Product1/2
  Gain/1 -> V_1s/1

== system ctrl_student_HIL/ControllerAndParanetrization/Controller1/Control parameterization/BacksteppingParameterization /Z_1 ==
  eta_hat : Inport
  p_d : Inport  Port=2
  "yaw " : Inport  Port=3
  Mux : Mux  Inputs=2
  Product : Product  Multiplication=Matrix(*)
  R Transposed : MATLAB Function  TreatAsAtomicUnit=on
  Reshape1 : Reshape  OutputDimensionality=Customize  OutputDimensions=[3,3]
  Reshape2 : Reshape  OutputDimensionality=Customize  OutputDimensions=[3,3]
  Reshape3 : Reshape  OutputDimensionality=Customize
  Rotation Matrix : MATLAB Function  TreatAsAtomicUnit=on
  Sum : Sum  Inputs=|+-
  z_1 : Outport
  R_T : Outport  Port=2
  wires:
  "yaw "/1 -> Reshape3/1, Mux/2
  p_d/1 -> Mux/1
  Sum/1 -> Product/2
  Rotation Matrix/1(R) -> Reshape2/1
  Product/1 -> z_1/1
  Mux/1 -> Sum/2
  R Transposed/1(R_T) -> Reshape1/1
  Reshape1/1 -> Product/1, R_T/1
  eta_hat/1 -> Sum/1
  Reshape2/1 -> R Transposed/1(R)
  Reshape3/1 -> Rotation Matrix/1(yaw)

== system ctrl_student_HIL/ControllerAndParanetrization/Controller1/Control parameterization/BacksteppingParameterization /alpha 1 ==
  z_1 : Inport
  eta_ds : Inport  Port=2
  U_s : Inport  Port=3
  R_T : Inport  Port=4
  Gain : Gain  Gain=-1
  "Kp " : Constant  Value=K1
  Product : Product  Multiplication=Matrix(*)
  Product1 : Product  Multiplication=Matrix(*)
  Product2 : Product  Multiplication=Matrix(*)
  Reshape : Reshape  OutputDimensionality=Customize  OutputDimensions=[3,1]
  Reshape1 : Reshape  OutputDimensionality=Customize
  Sum : Sum  Inputs=|++
  alpha1 : Outport
  wires:
  "Kp "/1 -> Gain/1
  Gain/1 -> Product/1
  z_1/1 -> Product/2
  Sum/1 -> alpha1/1
  Product/1 -> Sum/1
  Product1/1 -> Product2/2
  eta_ds/1 -> Reshape/1
  U_s/1 -> Reshape1/1
  Reshape/1 -> Product1/1
  Reshape1/1 -> Product1/2
  Product2/1 -> Sum/2
  R_T/1 -> Product2/1

== system ctrl_student_HIL/ControllerAndParanetrization/Controller1/Controller/Controller/alpha_1dott ==
  z_1 : Inport
  K_1 : Inport  Port=2
  eta_ds : Inport  Port=3
  R_T : Inport  Port=4
  U_s : Inport  Port=5
  s_dott : Inport  Port=6
  eta_dss : Inport  Port=7
  U_ss : Inport  Port=8
  nu : Inport  Port=9
  Demux1 : Demux  Outputs=3
  MATLAB Function : MATLAB Function  TreatAsAtomicUnit=on
  Terminator : Terminator
  Terminator1 : Terminator
  alpha_1dott : Outport
  wires:
  Demux1/1 -> Terminator/1
  Demux1/2 -> Terminator1/1
  nu/1 -> MATLAB Function/2(nu), Demux1/1
  Demux1/3 -> MATLAB Function/3(r)
  K_1/1 -> MATLAB Function/1(K_1)
  eta_ds/1 -> MATLAB Function/4(eta_ds)
  R_T/1 -> MATLAB Function/5(R_T)
  U_s/1 -> MATLAB Function/6(U_s)
  s_dott/1 -> MATLAB Function/7(s_dot)
  U_ss/1 -> MATLAB Function/9(U_ss)
  eta_dss/1 -> MATLAB Function/8(eta_dss)
  MATLAB Function/1(alpha_1dott) -> alpha_1dott/1
  z_1/1 -> MATLAB Function/10(z_1)

== system ctrl_student_HIL/ControllerAndParanetrization/PathParameterization/PathGenerization_Ellips/Path parametization /Subsystem ==
  Elipscenter_radi : Inport
  s : Inport  Port=2
  U_ref : Inport  Port=3
  MATLAB Function : MATLAB Function  TreatAsAtomicUnit=on
  Reshape1 : Reshape  OutputDimensionality=Customize  OutputDimensions=[2,1]
  Reshape2 : Reshape  OutputDimensionality=Customize  OutputDimensions=[3,1]
  Reshape3 : Reshape  OutputDimensionality=Customize  OutputDimensions=[3,1]
  Scope : Scope
      settings: YMin=0.05  YMax=0.4
  P_d : Outport
  Pd_s : Outport  Port=2
  eta_ds : Outport  Port=3
  eta_dss : Outport  Port=4
  U_ss : Outport  Port=5
  wires:
  MATLAB Function/1(pd) -> P_d/1
  Reshape1/1 -> Pd_s/1
  Elipscenter_radi/1 -> MATLAB Function/1(Elipscenter_radi)
  s/1 -> Scope/1, MATLAB Function/2(s)
  Reshape2/1 -> eta_ds/1
  MATLAB Function/2(pd_s) -> Reshape1/1
  MATLAB Function/3(eta_ds) -> Reshape2/1
  MATLAB Function/4(eta_dss) -> Reshape3/1
  Reshape3/1 -> eta_dss/1
  U_ref/1 -> MATLAB Function/3(U_ref)
  MATLAB Function/5(U_ss) -> U_ss/1

== system ctrl_student_HIL/ControllerAndParanetrization/PathParameterization/PathGenerization_Straight/Path parametization /Eta_ds ==
  s : Inport
  p_ds : Inport  Port=2
  Constant : Constant  Value=0
  Constant1 : Constant  Value=0
  Demux : Demux  Outputs=2
  MATLAB Function : MATLAB Function  TreatAsAtomicUnit=on
  MATLAB Function1 : MATLAB Function  Commented=on  TreatAsAtomicUnit=on
  Memory s : Memory  Commented=on
  Memory x_d : Memory  Commented=on
  Memory y_d : Memory  Commented=on
  Mux : Mux  Inputs=2
  eta_ds : Outport
  wires:
  MATLAB Function1/2(y_dd) -> Memory y_d/1
  Demux/1 -> MATLAB Function/1(x_d), MATLAB Function1/1(x_d)
  Mux/1 -> eta_ds/1
  Demux/2 -> MATLAB Function1/2(y_d), MATLAB Function/2(y_d)
  s/1 -> MATLAB Function1/3(s)
  p_ds/1 -> Mux/1, Demux/1
  MATLAB Function1/1(x_dd) -> Memory x_d/1
  Memory y_d/1 -> MATLAB Function1/5(y_dPrev)
  Memory x_d/1 -> MATLAB Function1/4(x_dPrev)
  Memory s/1 -> MATLAB Function1/6(s_Prev)
  MATLAB Function1/3(s1) -> Memory s/1
  MATLAB Function/1(eta_ds_yaw) -> Mux/2
  Constant/1 -> MATLAB Function/3(x_dd)
  Constant1/1 -> MATLAB Function/4(y_dd)

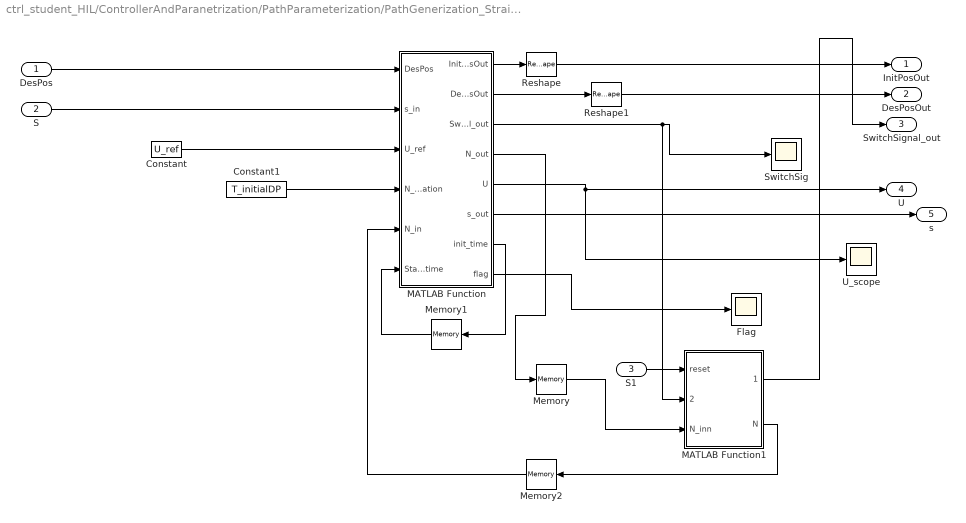
== system ctrl_student_HIL/ControllerAndParanetrization/PathParameterization/PathGenerization_Straight/Path parametization /Subsystem ==
  DesPos : Inport
  S : Inport  Port=2
  S1 : Inport  Port=3
  Constant : Constant  Value=U_ref
  Constant1 : Constant  Value=T_initialDP
  Flag : Scope
      settings: YMin=0  YMax=50  SaveName=ScopeData17
  MATLAB Function : MATLAB Function  TreatAsAtomicUnit=on
  MATLAB Function1 : MATLAB Function  TreatAsAtomicUnit=on
  Memory : Memory  X0=1
  Memory1 : Memory  X0=[0,0]
  Memory2 : Memory  X0=1
  Reshape : Reshape  OutputDimensionality=Customize  OutputDimensions=[2,1]
  Reshape1 : Reshape  OutputDimensionality=Customize  OutputDimensions=[2,1]
  SwitchSig : Scope
      settings: SaveName=ScopeData18
  "U_scope " : Scope
      settings: YMin=-1  YMax=1  SaveName=ScopeData16
  InitPosOut : Outport
  DesPosOut : Outport  Port=2
  SwitchSignal_out : Outport  Port=3
  U : Outport  Port=4
  s : Outport  Port=5
  wires:
  MATLAB Function/1(InitPosOut) -> Reshape/1
  MATLAB Function/2(DesPosOut) -> Reshape1/1
  DesPos/1 -> MATLAB Function/1(DesPos)
  S/1 -> MATLAB Function/2(s_in)
  Memory/1 -> MATLAB Function1/3(N_inn)
  MATLAB Function/4(N_out) -> Memory/1
  MATLAB Function/3(SwitchSignal_out) -> MATLAB Function1/2(SwitchSignal_inn), SwitchSig/1
  Reshape/1 -> InitPosOut/1
  Reshape1/1 -> DesPosOut/1
  Constant/1 -> MATLAB Function/3(U_ref)
  MATLAB Function/6(s_out) -> s/1
  MATLAB Function/5(U) -> "U_scope "/1, U/1
  Constant1/1 -> MATLAB Function/4(N_iteration)
  MATLAB Function/7(init_time) -> Memory1/1
  Memory1/1 -> MATLAB Function/6(Start_time)
  MATLAB Function/8(flag) -> Flag/1
  S1/1 -> MATLAB Function1/1(reset)
  MATLAB Function1/2(N) -> Memory2/1
  MATLAB Function1/1(SwitchSignal) -> SwitchSignal_out/1
  Memory2/1 -> MATLAB Function/5(N_in)

== matlab function ctrl_student_HIL/Deg2Rad ==
  data: deg input; rad output
function rad = fcn(deg)

rad=deg2rad(deg);

end

== matlab function ctrl_student_HIL/joystick/Contoller_Map1 ==
  data: current_mode input; glob_forces input; posSurge input; posSway input; posYaw input; tau_surge output; tau_sway output; tau_yaw output
function [tau_surge,tau_sway,tau_yaw] = fcn(current_mode,glob_forces,posSurge,posSway,posYaw)

if current_mode==2
    tau_surge=posSurge*glob_forces(1);
    tau_sway=0;
    tau_yaw=posYaw*glob_forces(4); 
else
    tau_surge=posSurge*glob_forces(1);
    tau_sway=posSway*glob_forces(2);
    tau_yaw=posYaw*glob_forces(3);
end

end

== matlab function ctrl_student_HIL/Noise generator/Downsample	signal/MATLAB Function ==
  data: f input; h input; i input; count output
function count = fcn(f,h,i)
%#codegen
sampling_time = 1/f;
if (i+1)*h >= sampling_time
    count = 0;
else
    count = i+1;
end

== matlab function ctrl_student_HIL/Rad2Deg ==
  data: deg output; rad input
function deg = fcn(rad)

deg=rad2deg(rad);

end

== matlab function ctrl_student_HIL/Noise generator/Sample & hold/MATLAB Function1 ==
  data: counter input; input input; hold input; output output
function output = fcn(counter,input,hold)
%#codegen

if counter == 0
    output = input;
else
    output = hold;
end

== matlab function ctrl_student_HIL/physics_model/kinematics ==
  data: nu input; eta_dot output; eta input
function eta_dot = CSE1_eta_dot(nu,eta)

psi = eta(3);

J = [cos(psi) -sin(psi) 0
     sin(psi) cos(psi)  0
     0        0         1];

eta_dot = J*nu;
end

== matlab function ctrl_student_HIL/ControllerAndParanetrization/PathParameterization/PathGenerization_Straight/Path parametization /Subsystem/MATLAB Function1 ==
  data: reset input; SwitchSignal output; N output; SwitchSignal_inn input; N_inn input
function [SwitchSignal,N] = fcn(reset,SwitchSignal_inn,N_inn)

if reset==1
    SwitchSignal=0;
    N=1;
else
    SwitchSignal=SwitchSignal_inn;
    N=N_inn;
end


end

== matlab function ctrl_student_HIL/joystick/Sel_Control_Mode ==
  data: previous_condition input; select input; current_mode output
function current_mode= fcn(previous_condition, select)

if select==1
    if previous_condition ==2
        current_mode=3;
    else
        current_mode=2;
    end
else
    current_mode=previous_condition;
end

end

== matlab function ctrl_student_HIL/safety zone /KillSwitch ==
  data: tau output; eta input; Kill_signal output; lim_2 input; tau_inn input; kill_inn input
function [tau,Kill_signal] = fcn(eta,lim_2,tau_inn,kill_inn)

if kill_inn==1;
    Kill_signal=1;
    %disp('Flag 3.0 KILL - previous kill');
else
    if eta(1)>=lim_2(1)
        Kill_signal=1;
        X=1;
        %disp('Flag 3.1 KILL - large x');
    elseif eta(1)<=lim_2(2)
        Kill_signal=1;
        X=1;
        %disp('Flag 3.2 KILL - small x');
    else
        Kill_signal=0;
        X=0;
    end %IF
    if eta(2)>=lim_2(3)
        Kill_signal=1;
        %disp('Flag 3.3 KILL - large y');
    elseif eta(2)<=lim_2(4)
        Kill_signal=1;
        %disp('Flag 3.4 KILL - small y');
    else
        if X==1
            Kill_signal=1;
        else
            Kill_signal=0; 
        end
        
    end %IF
end% IF

if Kill_signal==1
    tau=[0;0;0];
else
    tau=tau_inn;    
end %IF


end %Function

== matlab function ctrl_student_HIL/safety zone /MATLAB Function ==
  data: kill_signalInn input; kill_signal output; Comand input
function kill_signal = fcn(kill_signalInn,Comand)

if Comand==1
    kill_signal=0;
else
    kill_signal=kill_signalInn;
end

end

== matlab function ctrl_student_HIL/safety zone /Safety Act ==
  data: joyStick input; safetySig_1 input; safetySig_2 input; safetySig_3 input; safetySig_4 input; thrust_out output; vel input; switch_sig output; K input
function [thrust_out,switch_sig] = fcn(joyStick,safetySig_1,safetySig_2,safetySig_3,safetySig_4,vel,K)

switch_sig=0;
thrust_out=zeros(3,1);
%K=[1;1];    

    if safetySig_1 == 0 && safetySig_2 == 0 && safetySig_3 == 0 && safetySig_4 == 0   %Check to see if intervention is requiered
        
    switch_sig = 0; %Intervention is NOT requiered
    ThrustX=joyStick(1);
    ThrustY=joyStick(2);
       %disp('Flag 0.0 All OK - No safety sig');
    else
    switch_sig=1;   %Intervention IS requiered
    
        if  safetySig_1==1 || safetySig_2==1 %Problem in X dir
            %disp('Flag 1.0 Problem in x');
            if joyStick(1)==0 %Check if inputforce fore is zero or correct, (but the velocity might not be)
               %Perhaps a proprtional gain depending on the velocity?
               if vel(1)<0 && safetySig_2==1
                   ThrustX=K(1)*-vel(1);
                   %disp('Flag 1.1 (x - tau=0 - Negative vel + to low x pos -> thrust =-vel*K_1)');
               elseif vel(1)> 0 && safetySig_1==1
                   ThrustX=K(1)*-vel(1);
                   %disp('Flag 1.2 (x - tau=0 - Positive vel + to high x pos -> thrust =-vel*K_1)');
               else
                   ThrustX=K(1)*vel(1);
                   %disp('Flag 1.3 (x - tau=0 - Positive vel + to low x pos / Negative vel + to highx pos -> keep current trust)');
               end
                %thrust_out=[ThrustX;joyStick(2);joyStick(3)];
                
            elseif joyStick(1) >0 && safetySig_2==1     %X cord to small, but thrust right way
                ThrustX=joyStick(1);
                %thrust_out=[joyStick(1);joyStick(2);joyStick(3)];
                %disp('Flag 1.4 (x - Positive thrust + to low x post -> keep current trust)');
            elseif joyStick(1) <0 && safetySig_1==1     %X cord to large, but thrust right way
                ThrustX=joyStick(1);
                %thrust_out=[joyStick(1);joyStick(2);joyStick(3)];
                %disp('Flag 1.5 (x - Negative thrust + to high x post -> Keep current trust)');
            else
                ThrustX=-joyStick(1);
                %thrust_out=[-joyStick(1);joyStick(2);joyStick(3)];
                %disp('Flag 1.6 (x - Negative thrust + to low x post / Positive thrust + to high x post -> reverse trust)');
            end %If
        else
            ThrustX=joyStick(1);
        end %IF  
        
        if  safetySig_3==1 || safetySig_4==1 %Problem in X dir%Problem in Y dir
            %disp('Flag 2.0 Problem in y');
            if joyStick(2)==0 %Check if inputforce fore is zero or correct
                %Perhaps a proprtional gain depending on the velocity?  
                if vel(2)>0 && safetySig_3==1
                    ThrustY=K(2)*-vel(2);
                    %disp('Flag 2.1 (y - tau=0 - Negative vel + to low y pos -> thrust =-vel*K_2)');
                elseif vel(2)< 0 && safetySig_4==1
                    ThrustY=K(2)*-vel(2);
                    %disp('Flag 2.2 (y - tau=0 - Positive vel + to high y pos -> thrust =-vel*K_2)');
                else
                    ThrustY=K(2)*vel(2);
                    %disp('Flag 2.3 (y - tau=0 - Positive vel + to low y pos / Negative vel + to high y pos -> keep current trust)');
                end %IF
                %thrust_out=[joyStick(1);ThrustY;joyStick(3)];
                  
            elseif joyStick(2) >0 && safetySig_4==1     %Y cord to small
                ThrustY=joyStick(2);
                %thrust_out=[joyStick(1);joyStick(2);joyStick(3)];
                %disp('Flag 2.4 (y - Positive thrust + to low y post -> keep current trust)');
                
            elseif joyStick(2) <0 && safetySig_3==1     %Y cord to large
                ThrustY=joyStick(2);
                %thrust_out=[joyStick(1);joyStick(2);joyStick(3)];
                %disp('Flag 2.5 (y - Negative thrust + to high y post -> Keep current trust)');
                
            else
                ThrustY=-joyStick(2);
            %thrust_out=[joyStick(1);-joyStick(2);joyStick(3)];
            %disp('Flag 2.6 (y - Negative thrust + to low y post / Positive thrust + to high y post -> reverse trust)');
            
            end %IF
        else
            ThrustY=joyStick(2);
        end %IF
        
    end %IF
        thrust_out=[ThrustX;ThrustY;joyStick(3)];
end %Function

== matlab function ctrl_student_HIL/safety zone /safety check ==
  data: eta input; safety_sig_1 output; safety_sig_2 output; safety_sig_3 output; safety_sig_4 output; lim input
function [safety_sig_1,safety_sig_2,safety_sig_3,safety_sig_4]= fcn(eta,lim)


%safety_sig=[0;0;0;0];%orginal safety signal
%lim=[40.00;0;6.45;0];%space limitation [x_max;x_min;y_max;y_min]
if eta(1)>=lim(1)
    safety_sig_1 = 1;
    safety_sig_2= 0;
elseif eta(1)<=lim(2)
    safety_sig_2 = 1;
    safety_sig_1=0;
else
    safety_sig_1 = 0;
    safety_sig_2 = 0;
end
if eta(2)>lim(3)
    safety_sig_3 = 1;
    safety_sig_4 = 0;
elseif eta(2)<lim(4)
    safety_sig_4 = 1;
    safety_sig_3 = 0;

else
    safety_sig_3 = 0;
    safety_sig_4 = 0;
end
% safety_sig_1=safety_sig(1);
% safety_sig_2=safety_sig(2);
%safety_sig_3=safety_sig(3);
%safety_sig_4=safety_sig(4);

end

== matlab function ctrl_student_HIL/ControllerAndParanetrization/Controller1/Control parameterization/BacksteppingParameterization /V_1s/MATLAB Function ==
  data: z_1 input; z_1T output
function z_1T = fcn(z_1)

z_1T=z_1';
end

== matlab function ctrl_student_HIL/Dropout_simulator/MATLAB Function ==
  data: X_in input; X_out output; Y_out output; Yaw_out output; Y_in input; Yaw_in input; Dropoutsignal input; X_prev input; Y_prev input; Yaw_prev input
function [X_out,Y_out,Yaw_out] = fcn(X_in,Y_in,Yaw_in,Dropoutsignal,X_prev,Y_prev,Yaw_prev)
X_out=-1;
Y_out=-1;
Yaw_out=-1;


switch Dropoutsignal
    case 0
        X_out =X_in;
        Y_out=Y_in;
        Yaw_out=Yaw_in;
        
    case 1        
        X_out =X_prev;
        Y_out=Y_prev;
        Yaw_out=Yaw_prev;
end


end

== matlab function ctrl_student_HIL/ControllerAndParanetrization/Controller1/Control parameterization/BacksteppingParameterization /V_1s/MATLAB Function1 ==
  data: R input; R_T output
function R_T = fcn(R)

R_T=transpose(R);

end

== matlab function ctrl_student_HIL/ControllerAndParanetrization/Controller1/Controller/Controller/MATLAB Function ==
  data: u input; D output; v input; r input
function D = fcn(u,v,r)
%% Damping coefficients
% Comments at the end of the lines indicate the old values used.
X_u		= -0.6555;		X_v		= 0;
X_uu 	= 0.3545;		X_vv	= -2.443;
X_uuu 	= -3.787;		X_vvv	= 0;

Y_v		= -1.33; 			Y_r		= -7.250; % Y_r
Y_vv	= -2.776;			Y_rr	= -3.450; % Y_rr
Y_vvv	= -64.91;			Y_rrr	= 0;
						
Y_rv	= -0.805;			Y_vr	= -0.845; % Y_rv, Y_vr

N_v		= 0;				N_r		= -1.900; % N_r
N_vv	= -0.2088;			N_rr	= -0.750; % N_rr
N_vvv	= 0;				N_rrr	= 0;
N_rv	= 0.130;			N_vr	= 0.080; % N_rv, N_vr
d_11 = -X_u - X_uu*u - X_uuu*u^2;
d_22 = -Y_v - Y_vv*v - Y_vvv*v^2 - Y_rv*abs(r);
d_33 = -N_r - N_rr*abs(r) - N_rrr*r^2 - N_vr*abs(v); % using abs(r)

d_12 = -X_v - X_vv*v - X_vvv*v^2;
d_23 = -Y_r - Y_rr*abs(r) - Y_rrr*r^2 - Y_vr*abs(v);
d_32 = -N_v - N_vv*v - N_vvv*v^2 - N_rv*abs(r);

D    = [d_11 0    0
        0    d_22 d_23
        0    d_32 d_33];
end

== matlab function ctrl_student_HIL/ControllerAndParanetrization/Controller1/Controller/Controller/MATLAB Function1 ==
  data: m input; M output
function M = fcn(m)
%% MATRICES

   I_z  =  1.7600;   x_g = 0.0375;       % x_g  =  0.0460; % Table B.1


%% Added mass
X_ud  =     -2.0;											% Table B.1
					Y_vd =     -1.0;	N_vd =    -0.0;		% Table B.1 guestimate
					Y_rd =      -0.0;	N_rd =    -1.0;		% Table B.1

%% Total mass matrix
m_11 = m-X_ud;
m_22 = m-Y_vd;
m_23 = m*x_g-Y_rd;
m_32 = m*x_g-N_vd;
m_33 = I_z-N_rd;

M    = [m_11 0    0
        0    m_22 m_23
        0    m_32 m_33];
end
